simulink model "example_main_NDI_f16"  (R2020a)
settings: Solver=ode4  StartTime=0.0  StopTime=75  FixedStep=0.01  RelTol=1e-3
PreLoadFcn:
  | PreLoadFcn
values from neighbouring files (symbols this model uses):
  g = 32.17    [PreLoadFcn.m]
  N = [ 1      0     0.25 ... (first row only)    [PreLoadFcn.m]
  state0 = [IC.npos IC.epos IC.alt IC.q0 IC.q1 IC.q2 IC.q3  IC.p IC.q IC.r IC.alpha IC.beta IC.mu IC.Vt IC.chi IC.gamma]    [PreLoadFcn.m]
undefined symbols (not defined in the file or in its folder): Aactuator, ac, AeroCoeff, EngineTable, ft, IC, kg, m, Newton, PIController, Raphson, s, sigbuilder_block, slug
libraries: aerolibconvert2 x19, simulink x13, sharedutil x1
(part 2 of 6)

== system example_main_NDI_f16/Environment/ISP  ==
  note: 1 T
      | 2 a (Speed of sound)
      | 3 P
      | 4 rho
      | 5 g
      | 6 mu (Coefficient of viscosity)
  In Bus Element : Inport  PortName=PlantData  Element=Vt
  In Bus Element1 : Inport  PortName=PlantData  Element=altitude
  Demux : Demux  Outputs=[1,1,1,1,1,1]
      settings: DisplayOption=none
  Density Conversion : aerolibconvert2/Density Conversion  IU=kg/m^3  OU=slug/ft^3
      settings: SourceProductBaseCode=AE
  Divide1 : Product  Inputs=*/
  Length Conversion : aerolibconvert2/Length Conversion  IU=ft  OU=m
  MATLAB Function : MATLAB Function  TreatAsAtomicUnit=on
  Product : Product
  Square : Math  Operator=square  SignedPower=on  SaturateOnIntegerOverflow=on
  Velocity Conversion : aerolibconvert2/Velocity Conversion  IU=m/s  OU=ft/s
  r2d1 : Gain  Gain=0.5  SaturateOnIntegerOverflow=on  OutDataTypeStr=Inherit: Same as input  ParamDataTypeStr=Inherit: Same as input
  r2d2 : Gain  Gain=-1  SaturateOnIntegerOverflow=on  OutDataTypeStr=Inherit: Same as input  ParamDataTypeStr=Inherit: Same as input
  P(HPa) : Outport  VectorParamsAs1DForOutWhenUnconnected=off
  rho(kg/m^3) : Outport  Port=2  VectorParamsAs1DForOutWhenUnconnected=off
  qbar (lbf/ft^2) : Outport  Port=3  VectorParamsAs1DForOutWhenUnconnected=off
  "Mach " : Outport  Port=4  VectorParamsAs1DForOutWhenUnconnected=off
  T(K) : Outport  Port=5  VectorParamsAs1DForOutWhenUnconnected=off
  g (m/s^2) : Outport  Port=6  VectorParamsAs1DForOutWhenUnconnected=off
  mu : Outport  Port=7  VectorParamsAs1DForOutWhenUnconnected=off
  wires:
  MATLAB Function/1(ISP_output) -> Demux/1
  Length Conversion/1 -> MATLAB Function/1(h)
  Velocity Conversion/1 -> Divide1/2
  Density Conversion/1 -> Product/2  "rho(slugs/ft^3)"
  Demux/4 -> Density Conversion/1, rho(kg/m^3)/1  "rho(kg/m^3)"
  Demux/2 -> Velocity Conversion/1  "a(m/s)"
  Demux/1 -> T(K)/1  "T(K)"
  Divide1/1 -> "Mach "/1
  Demux/5 -> g (m/s^2)/1  "g (m/s^2)"
  Demux/6 -> mu/1  "mu"
  Product/1 -> r2d1/1
  Square/1 -> Product/1
  In Bus Element/1 -> Divide1/1, Square/1  "Vt (ft/s)"
  Demux/3 -> P(HPa)/1  "P(Pa)"
  r2d2/1 -> Length Conversion/1  "H(ft)"
  r2d1/1 -> qbar (lbf/ft^2)/1  "qbar (lbf/ft^2)"
  In Bus Element1/1 -> r2d2/1

== system example_main_NDI_f16/F-16 Vehicle Systems Model/6.4.3加裝向量噴嘴以及減速版打開30度模擬著陸速度為200， 上下偏轉向量噴嘴權重值為4，75S (附錄B須調整權重值: 2、4、8、16) ==
  Demux : Demux  Tag=STV Demux  Outputs=5
      settings: DisplayOption=none
  FromWs : FromWorkspace  Tag=STV FromWs  VariableName=tuvar
      SigBuilderData=|
      | common.afterFinalStr = 'Extrapolate'
      | common.sampleTime = 0
      | dataSet.timeRange = [0 90]
      | dataSet.name = 'Group 1'
      | sbobj.Groups.Name = 'Group 1'
      | sbobj.Groups.Signals(1).Name = 'Vt (ft/s)'
      | sbobj.Groups.Signals(1).XData = [0 5 6.2 7.35 8.3 9.05 10.05 11.2 13.1 14.75 15 16.85 18.75 19.63 20 22.2 23.5 25 26.65 30 31.65 40 50 60 75 80 90]
      | sbobj.Groups.Signals(1).YData = [287 287 286.6 286 285 284.6 283.9 283.4 281.8 279.8 279.4 277 274.8 273.8 273.3 270.3 268.6 266.55 263.7 260 258 250 240 227 200 226 210]
      | sbobj.Groups.Signals(2).Name = 'y (ft)'
      | sbobj.Groups.Signals(2).XData = [0 90]
      | sbobj.Groups.Signals(2).YData = [0 0]
      | sbobj.Groups.Signals(3).Name = 'h (ft)'
      | sbobj.Groups.Signals(3).XData = [0 55 75 90]
      | sbobj.Groups.Signals(3).YData = [993 93 0 0]
      | sbobj.Groups.Signals(4).Name = 'speed brake (deg)'
      | sbobj.Groups.Signals(4).XData = [0 90]
      | sbobj.Groups.Signals(4).YData = [30 30]
      | sbobj.Groups.Signals(5).Name = 'LandingGear_position'
      | sbobj.Groups.Signals(5).XData = [0 90]
      | sbobj.Groups.Signals(5).YData = [1 1]
      | sbobj.Groups.TimeRange = [0 90]
  Vt (ft/s) : Outport  Tag=STV Outport  VectorParamsAs1DForOutWhenUnconnected=off
  y (ft) : Outport  Tag=STV Outport  Port=2  VectorParamsAs1DForOutWhenUnconnected=off
  h (ft) : Outport  Tag=STV Outport  Port=3  VectorParamsAs1DForOutWhenUnconnected=off
  speed brake (deg) : Outport  Tag=STV Outport  Port=4
  LandingGear_position : Outport  Tag=STV Outport  Port=5
  wires:
  FromWs/1 -> Demux/1
  Demux/1 -> Vt (ft/s)/1
  Demux/2 -> y (ft)/1
  Demux/3 -> h (ft)/1
  Demux/4 -> speed brake (deg)/1
  Demux/5 -> LandingGear_position/1

== system example_main_NDI_f16/F-16 Vehicle Systems Model/6.4.3加裝向量噴嘴以及減速版打開40度模擬著陸速度為200， 上下偏轉向量噴嘴權重值為5.5，75S ==
  Demux : Demux  Tag=STV Demux  Outputs=5
      settings: DisplayOption=none
  FromWs : FromWorkspace  Tag=STV FromWs  VariableName=tuvar
      SigBuilderData=|
      | common.afterFinalStr = 'Extrapolate'
      | common.sampleTime = 0
      | dataSet.timeRange = [0 80]
      | dataSet.name = 'Group 1'
      | sbobj.Groups.Name = 'Group 1'
      | sbobj.Groups.Signals(1).Name = 'Vt (ft/s)'
      | sbobj.Groups.Signals(1).XData = [0 5 6.2 7.35 8.3 9.05 10.05 11.2 13.1 14.75 15 16.85 18.75 19.63 20 22.2 23.5 25 26.65 33 36.65 45 55 65 75 80]
      | sbobj.Groups.Signals(1).YData = [287 287 286.6 286 285 284.6 283.9 283.4 281.8 279.8 279.4 277 274.8 273.8 273.3 270.3 268.6 266.55 264 258 255.5 246 234 220 200 214]
      | sbobj.Groups.Signals(2).Name = 'y (ft)'
      | sbobj.Groups.Signals(2).XData = [0 80]
      | sbobj.Groups.Signals(2).YData = [0 0]
      | sbobj.Groups.Signals(3).Name = 'h (ft)'
      | sbobj.Groups.Signals(3).XData = [0 55 75 80]
      | sbobj.Groups.Signals(3).YData = [993 93 0 0]
      | sbobj.Groups.Signals(4).Name = 'speed brake (deg)'
      | sbobj.Groups.Signals(4).XData = [0 80]
      | sbobj.Groups.Signals(4).YData = [40 40]
      | sbobj.Groups.Signals(5).Name = 'LandingGear_position'
      | sbobj.Groups.Signals(5).XData = [0 80]
      | sbobj.Groups.Signals(5).YData = [1 1]
      | sbobj.Groups.TimeRange = [0 80]
  Vt (ft/s) : Outport  Tag=STV Outport  VectorParamsAs1DForOutWhenUnconnected=off
  y (ft) : Outport  Tag=STV Outport  Port=2  VectorParamsAs1DForOutWhenUnconnected=off
  h (ft) : Outport  Tag=STV Outport  Port=3  VectorParamsAs1DForOutWhenUnconnected=off
  speed brake (deg) : Outport  Tag=STV Outport  Port=4  VectorParamsAs1DForOutWhenUnconnected=off
  LandingGear_position : Outport  Tag=STV Outport  Port=5  VectorParamsAs1DForOutWhenUnconnected=off
  wires:
  FromWs/1 -> Demux/1
  Demux/1 -> Vt (ft/s)/1
  Demux/2 -> y (ft)/1
  Demux/3 -> h (ft)/1
  Demux/4 -> speed brake (deg)/1
  Demux/5 -> LandingGear_position/1

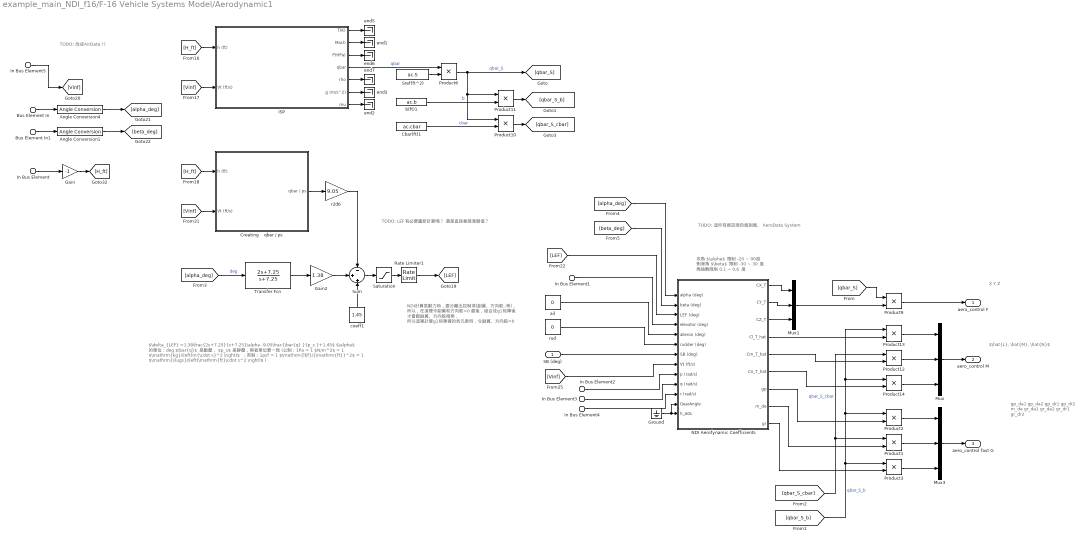
== system example_main_NDI_f16/F-16 Vehicle Systems Model/Aerodynamic1 ==
  note: NDI計算氣動力時，要分離出控制項(副翼、方向舵..等)，
      | 所以，在這裡令副翼和方向舵=0
      | 最後，組合成g1矩陣後 才會跟副翼、方向舵相乘，
      | 所以這裡計算g1矩陣裡的各元素時，令副翼、方向舵=0
  note: TODO: LEF有必要重新計算嗎？
      | 還是直接拿感測器值？
  note: X
      | Y
      | Z
  note: gp_da1
      | gp_da2
      | gp_dr1
      | gp_dr2
      | m_de
      | gr_da1
      | gr_da2
      | gr_dr1
      | gr_dr2
  note: $\delta_{LEF} =1.38\frac{2s+7.25}{s+7.25}\alpha -9.05\frac{\bar{q} }{p_s }+1.45$
      | $\alpha$ 的單位：deg
      | $\bar{q}$ 是動壓， $p_s$ 是靜壓，兩者單位要一致 (公制：1Pa = 1 $N/m^2$ = 1 $\mathrm{kg}/\left(m{\cdot s}^2 \right)$ ；英制：1psf = 1 $\mathrm{lbf}/{\mathrm{ft}}^2$ = 1 $\mathrm{slugs}/\left(\mathrm{ft}\cdot s^2 \right)$ )
  note: $\hat{L}, \hat{M}, \hat{N}$
  note: TODO: 這所有資訊源自感測器、
      | AeroData System
  note: TODO: 改成AirData !?
  note: 攻角 $\alpha$ 限制 -20 ~ 90度
      | 側滑角 $\beta$ 限制 -30 ~ 30 度
      | 馬赫數限制 0.1 ~ 0.6 度
  SB (deg) : Inport  Unit=deg
  In Bus Element : Inport  Port=2  PortName=PlantData  Element=altitude
  In Bus Element1 : Inport  Port=2  PortName=PlantData  Element=AeroActBus.Elevator_deg
  In Bus Element2 : Inport  Port=2  PortName=PlantData  Element=p
  In Bus Element3 : Inport  Port=2  PortName=PlantData  Element=q
  In Bus Element4 : Inport  Port=2  PortName=PlantData  Element=r
  In Bus Element5 : Inport  Port=2  PortName=PlantData  Element=Vt
  Bus Element In : Inport  Port=3  PortName=AirData  Element=alpha
  Bus Element In1 : Inport  Port=3  PortName=AirData  Element=beta
  Angle Conversion1 : aerolibconvert2/Angle Conversion  IU=rad  OU=deg
  Angle Conversion4 : aerolibconvert2/Angle Conversion  IU=rad  OU=deg
  Cbar(ft)1 : Constant  Value=ac.cbar
  Creating    qbar / ps : Subsystem
  Gain : Gain  Gain=-1
  Gain2 : Gain  Gain=1.38  SaturateOnIntegerOverflow=on  OutDataTypeStr=Inherit: Same as input  ParamDataTypeStr=Inherit: Same as input
  Ground : Ground
  "ISP " : Subsystem
  Mux : Mux  Inputs=3
  Mux1 : Mux  Inputs=3
  Mux3 : Mux  Inputs=3
  NDI Aerofynamic Coefficients : Subsystem
  Product{1..3,6,9..14} (10 alike) : Product
  Rate Limiter1 : RateLimiter  RisingSlewLimit=Aactuator.LEF.RateLimitUpper  FallingSlewLimit=Aactuator.LEF.RateLimitLower  SampleTimeMode=inherited  InitialCondition=Aactuator.LEF.IntegratorInitial
  Saturation : Saturate  UpperLimit=Aactuator.LEF.AngleLimitUpper  LowerLimit=Aactuator.LEF.AngleLimitLower
  Sref(ft^2) : Constant  Value=ac.S
  Sum : Sum  Inputs=-|+|+  InputSameDT=on  SaturateOnIntegerOverflow=on  OutDataTypeStr=Inherit: Same as first input
  Transfer Fcn : TransferFcn  Numerator=[2 7.25]  Denominator=[1 7.25]
  ail : Constant  Value=0
  b(ft)1 : Constant  Value=ac.b
  coeff1 : Constant  Value=1.45
  end{1..3,5..7} (6 alike) : Terminator
  r2d6 : Gain  Gain=9.05  SaturateOnIntegerOverflow=on  OutDataTypeStr=Inherit: Same as input  ParamDataTypeStr=Inherit: Same as input
  rud : Constant  Value=0
  aero_control F : Outport  VectorParamsAs1DForOutWhenUnconnected=off
  aero_control M : Outport  Port=2  VectorParamsAs1DForOutWhenUnconnected=off
  aero_control fast G : Outport  Port=3  VectorParamsAs1DForOutWhenUnconnected=off
  wires:
  [Vinf] -> "ISP "/2(Vt (ft/s))
  "ISP "/2("Mach ") -> end1/1
  "ISP "/7(mu) -> end2/1
  "ISP "/6(g (m/s^2)) -> end3/1
  "ISP "/5(rho) -> end7/1
  "ISP "/4("qbar ") -> Product6/1  "qbar"
  "ISP "/3(P(HPa)) -> end6/1
  "ISP "/1(T(K)) -> end5/1
  r2d6/1 -> Sum/1
  Creating    qbar / ps/1(qbar / ps) -> r2d6/1
  [alpha_deg] -> Transfer Fcn/1  "deg"
  [Vinf] -> Creating    qbar / ps/2(Vt (ft/s))
  coeff1/1 -> Sum/3
  [H_ft] -> Creating    qbar / ps/1(h (ft))
  [H_ft] -> "ISP "/1(h (ft))
  Sum/1 -> Saturation/1
  Saturation/1 -> Rate Limiter1/1
  Rate Limiter1/1 -> [LEF]
  Transfer Fcn/1 -> Gain2/1
  In Bus Element/1 -> Gain/1
  Gain/1 -> [H_ft]
  Cbar(ft)1/1 -> Product10/2  "cbar"
  b(ft)1/1 -> Product11/2  "b"
  Sref(ft^2)/1 -> Product6/2
  Product10/1 -> [qbar_S_cbar]
  Product6/1 -> Product11/1, Product10/1, [qbar_S]  "qbar_S"
  Product11/1 -> [qbar_S_b]
  [qbar_S] -> Product9/1
  Product9/1 -> aero_control F/1
  Product12/1 -> Mux/2
  Product13/1 -> Mux/1
  Product14/1 -> Mux/3
  Mux/1 -> aero_control M/1
  NDI Aerofynamic Coefficients/4(Cl_T_hat) -> Product13/2
  NDI Aerofynamic Coefficients/5(Cm_T_hat) -> Product12/2
  NDI Aerofynamic Coefficients/6(Cn_T_hat) -> Product14/2
  NDI Aerofynamic Coefficients/1(CX_T) -> Mux1/1
  NDI Aerofynamic Coefficients/2(CY_T) -> Mux1/2
  NDI Aerofynamic Coefficients/3(CZ_T) -> Mux1/3
  Mux1/1 -> Product9/2
  [qbar_S_b] -> Product13/1, Product14/1, Product2/1, Product3/1  "qbar_S_b"
  Product3/1 -> Mux3/3
  Product1/1 -> Mux3/2
  Product2/1 -> Mux3/1
  NDI Aerofynamic Coefficients/7(gp) -> Product2/2
  [qbar_S_cbar] -> Product12/1, Product1/1  "qbar_S_cbar"
  NDI Aerofynamic Coefficients/9(gr) -> Product3/2
  NDI Aerofynamic Coefficients/8(m_de) -> Product1/2
  Mux3/1 -> aero_control fast G/1
  [Vinf] -> NDI Aerofynamic Coefficients/8(Vt (ft/s))
  SB (deg)/1 -> NDI Aerofynamic Coefficients/7(SB (deg))
  [LEF] -> NDI Aerofynamic Coefficients/3(LEF (deg))
  rud/1 -> NDI Aerofynamic Coefficients/6(rudder (deg))
  ail/1 -> NDI Aerofynamic Coefficients/5(alieron (deg))
  In Bus Element1/1 -> NDI Aerofynamic Coefficients/4(elevator (deg))
  [beta_deg] -> NDI Aerofynamic Coefficients/2(beta (deg))
  [alpha_deg] -> NDI Aerofynamic Coefficients/1(alpha (deg))
  In Bus Element2/1 -> NDI Aerofynamic Coefficients/9(p (rad/s))
  In Bus Element3/1 -> NDI Aerofynamic Coefficients/10(q (rad/s))
  In Bus Element4/1 -> NDI Aerofynamic Coefficients/11(r (rad/s))
  Ground/1 -> NDI Aerofynamic Coefficients/12(GearAngle), NDI Aerofynamic Coefficients/13(h_AGL)
  Gain2/1 -> Sum/2
  Bus Element In/1 -> Angle Conversion4/1
  Angle Conversion4/1 -> [alpha_deg]
  Angle Conversion1/1 -> [beta_deg]
  Bus Element In1/1 -> Angle Conversion1/1
  In Bus Element5/1 -> [Vinf]

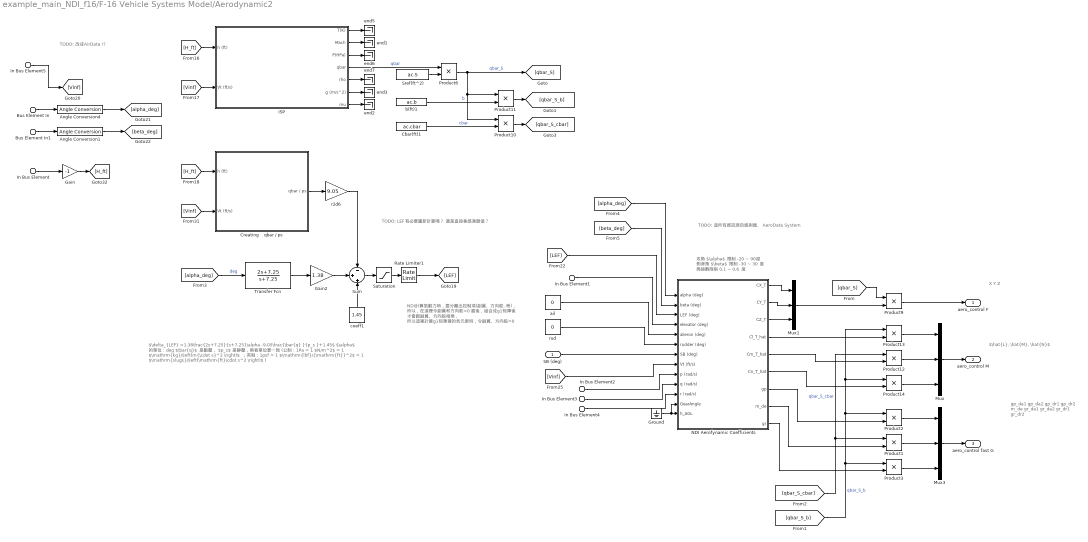
== system example_main_NDI_f16/F-16 Vehicle Systems Model/Aerodynamic2 ==
  note: NDI計算氣動力時，要分離出控制項(副翼、方向舵..等)，
      | 所以，在這裡令副翼和方向舵=0
      | 最後，組合成g1矩陣後 才會跟副翼、方向舵相乘，
      | 所以這裡計算g1矩陣裡的各元素時，令副翼、方向舵=0
  note: TODO: LEF有必要重新計算嗎？
      | 還是直接拿感測器值？
  note: X
      | Y
      | Z
  note: gp_da1
      | gp_da2
      | gp_dr1
      | gp_dr2
      | m_de
      | gr_da1
      | gr_da2
      | gr_dr1
      | gr_dr2
  note: $\delta_{LEF} =1.38\frac{2s+7.25}{s+7.25}\alpha -9.05\frac{\bar{q} }{p_s }+1.45$
      | $\alpha$ 的單位：deg
      | $\bar{q}$ 是動壓， $p_s$ 是靜壓，兩者單位要一致 (公制：1Pa = 1 $N/m^2$ = 1 $\mathrm{kg}/\left(m{\cdot s}^2 \right)$ ；英制：1psf = 1 $\mathrm{lbf}/{\mathrm{ft}}^2$ = 1 $\mathrm{slugs}/\left(\mathrm{ft}\cdot s^2 \right)$ )
  note: $\hat{L}, \hat{M}, \hat{N}$
  note: TODO: 這所有資訊源自感測器、
      | AeroData System
  note: TODO: 改成AirData !?
  note: 攻角 $\alpha$ 限制 -20 ~ 90度
      | 側滑角 $\beta$ 限制 -30 ~ 30 度
      | 馬赫數限制 0.1 ~ 0.6 度
  SB (deg) : Inport  Unit=deg
  In Bus Element : Inport  Port=2  PortName=PlantData  Element=altitude
  In Bus Element1 : Inport  Port=2  PortName=PlantData  Element=AeroActBus.Elevator_deg
  In Bus Element2 : Inport  Port=2  PortName=PlantData  Element=p
  In Bus Element3 : Inport  Port=2  PortName=PlantData  Element=q
  In Bus Element4 : Inport  Port=2  PortName=PlantData  Element=r
  In Bus Element5 : Inport  Port=2  PortName=PlantData  Element=Vt
  Bus Element In : Inport  Port=3  PortName=AirData  Element=alpha_c
  Bus Element In1 : Inport  Port=3  PortName=AirData  Element=beta_c
  Angle Conversion1 : aerolibconvert2/Angle Conversion  IU=rad  OU=deg
  Angle Conversion4 : aerolibconvert2/Angle Conversion  IU=rad  OU=deg
  Cbar(ft)1 : Constant  Value=ac.cbar
  Creating    qbar / ps : Subsystem
  Gain : Gain  Gain=-1
  Gain2 : Gain  Gain=1.38  SaturateOnIntegerOverflow=on  OutDataTypeStr=Inherit: Same as input  ParamDataTypeStr=Inherit: Same as input
  Ground : Ground
  "ISP " : Subsystem
  Mux : Mux  Inputs=3
  Mux1 : Mux  Inputs=3
  Mux3 : Mux  Inputs=3
  NDI Aerofynamic Coefficients : Subsystem
  Product{1..3,6,9..14} (10 alike) : Product
  Rate Limiter1 : RateLimiter  RisingSlewLimit=Aactuator.LEF.RateLimitUpper  FallingSlewLimit=Aactuator.LEF.RateLimitLower  SampleTimeMode=inherited  InitialCondition=Aactuator.LEF.IntegratorInitial
  Saturation : Saturate  UpperLimit=Aactuator.LEF.AngleLimitUpper  LowerLimit=Aactuator.LEF.AngleLimitLower
  Sref(ft^2) : Constant  Value=ac.S
  Sum : Sum  Inputs=-|+|+  InputSameDT=on  SaturateOnIntegerOverflow=on  OutDataTypeStr=Inherit: Same as first input
  Transfer Fcn : TransferFcn  Numerator=[2 7.25]  Denominator=[1 7.25]
  ail : Constant  Value=0
  b(ft)1 : Constant  Value=ac.b
  coeff1 : Constant  Value=1.45
  end{1..3,5..7} (6 alike) : Terminator
  r2d6 : Gain  Gain=9.05  SaturateOnIntegerOverflow=on  OutDataTypeStr=Inherit: Same as input  ParamDataTypeStr=Inherit: Same as input
  rud : Constant  Value=0
  aero_control F : Outport  VectorParamsAs1DForOutWhenUnconnected=off
  aero_control M : Outport  Port=2  VectorParamsAs1DForOutWhenUnconnected=off
  aero_control fast G : Outport  Port=3  VectorParamsAs1DForOutWhenUnconnected=off
  wires:
  [Vinf] -> "ISP "/2(Vt (ft/s))
  "ISP "/2("Mach ") -> end1/1
  "ISP "/7(mu) -> end2/1
  "ISP "/6(g (m/s^2)) -> end3/1
  "ISP "/5(rho) -> end7/1
  "ISP "/4("qbar ") -> Product6/1  "qbar"
  "ISP "/3(P(HPa)) -> end6/1
  "ISP "/1(T(K)) -> end5/1
  r2d6/1 -> Sum/1
  Creating    qbar / ps/1(qbar / ps) -> r2d6/1
  [alpha_deg] -> Transfer Fcn/1  "deg"
  [Vinf] -> Creating    qbar / ps/2(Vt (ft/s))
  coeff1/1 -> Sum/3
  [H_ft] -> Creating    qbar / ps/1(h (ft))
  [H_ft] -> "ISP "/1(h (ft))
  Sum/1 -> Saturation/1
  Saturation/1 -> Rate Limiter1/1
  Rate Limiter1/1 -> [LEF]
  Transfer Fcn/1 -> Gain2/1
  In Bus Element/1 -> Gain/1
  Gain/1 -> [H_ft]
  Cbar(ft)1/1 -> Product10/2  "cbar"
  b(ft)1/1 -> Product11/2  "b"
  Sref(ft^2)/1 -> Product6/2
  Product10/1 -> [qbar_S_cbar]
  Product6/1 -> Product11/1, Product10/1, [qbar_S]  "qbar_S"
  Product11/1 -> [qbar_S_b]
  [qbar_S] -> Product9/1
  Product9/1 -> aero_control F/1
  Product12/1 -> Mux/2
  Product13/1 -> Mux/1
  Product14/1 -> Mux/3
  Mux/1 -> aero_control M/1
  NDI Aerofynamic Coefficients/4(Cl_T_hat) -> Product13/2
  NDI Aerofynamic Coefficients/5(Cm_T_hat) -> Product12/2
  NDI Aerofynamic Coefficients/6(Cn_T_hat) -> Product14/2
  NDI Aerofynamic Coefficients/1(CX_T) -> Mux1/1
  NDI Aerofynamic Coefficients/2(CY_T) -> Mux1/2
  NDI Aerofynamic Coefficients/3(CZ_T) -> Mux1/3
  Mux1/1 -> Product9/2
  [qbar_S_b] -> Product13/1, Product14/1, Product2/1, Product3/1  "qbar_S_b"
  Product3/1 -> Mux3/3
  Product1/1 -> Mux3/2
  Product2/1 -> Mux3/1
  NDI Aerofynamic Coefficients/7(gp) -> Product2/2
  [qbar_S_cbar] -> Product12/1, Product1/1  "qbar_S_cbar"
  NDI Aerofynamic Coefficients/9(gr) -> Product3/2
  NDI Aerofynamic Coefficients/8(m_de) -> Product1/2
  Mux3/1 -> aero_control fast G/1
  [Vinf] -> NDI Aerofynamic Coefficients/8(Vt (ft/s))
  SB (deg)/1 -> NDI Aerofynamic Coefficients/7(SB (deg))
  [LEF] -> NDI Aerofynamic Coefficients/3(LEF (deg))
  rud/1 -> NDI Aerofynamic Coefficients/6(rudder (deg))
  ail/1 -> NDI Aerofynamic Coefficients/5(alieron (deg))
  In Bus Element1/1 -> NDI Aerofynamic Coefficients/4(elevator (deg))
  [beta_deg] -> NDI Aerofynamic Coefficients/2(beta (deg))
  [alpha_deg] -> NDI Aerofynamic Coefficients/1(alpha (deg))
  In Bus Element2/1 -> NDI Aerofynamic Coefficients/9(p (rad/s))
  In Bus Element3/1 -> NDI Aerofynamic Coefficients/10(q (rad/s))
  In Bus Element4/1 -> NDI Aerofynamic Coefficients/11(r (rad/s))
  Ground/1 -> NDI Aerofynamic Coefficients/12(GearAngle), NDI Aerofynamic Coefficients/13(h_AGL)
  Gain2/1 -> Sum/2
  Bus Element In/1 -> Angle Conversion4/1
  Angle Conversion4/1 -> [alpha_deg]
  Angle Conversion1/1 -> [beta_deg]
  Bus Element In1/1 -> Angle Conversion1/1
  In Bus Element5/1 -> [Vinf]

== system example_main_NDI_f16/F-16 Vehicle Systems Model/Iteration Algorithm V chi gamma ==
  note: $\mu_c ={\mathrm{tan}}^{-1} {\left(\frac{V_T {\chi^˙ }_{des} \mathrm{cos}\gamma }{V_T {\gamma^˙ }_{des} +g\mathrm{cos}\gamma }\right)}$
  note: $\alpha_c ={\mathrm{tan}}^{-1} {\left(\frac{-L+mV_T {\chi^˙ }_{des} \mathrm{cos}\gamma \mathrm{sin}\mu_c +mV_T {\gamma^˙ }_{des} \mathrm{cos}\mu_c +mg\mathrm{cos}\gamma \mathrm{cos}\mu_c }{m{\dot{V} }_{T_{des} } +D+mg\mathrm{sin}\gamma }\right)}$
  note: $T_c =\frac{1}{\mathrm{cos}\alpha_c }{\left(m{\dot{V} }_{T_{des} } +D+mg\mathrm{sin}\gamma \right)}$
  alpha_c : Inport
  aero F : Inport  Port=2
  Vt,chi,gamma dot desire : Inport  Port=3
  beta_cmd : Inport  Port=4
  gravity : Inport  Port=5
  In Bus Element4 : Inport  Port=6  PortName=AirData  Element=Vt
  In Bus Element5 : Inport  Port=6  PortName=AirData  Element=gamma
  Drag_c : Fcn  Expr=-u(4)*cos(u(2))*cos(u(3))-u(5)*sin(u(3))-u(6)*sin(u(2))*cos(u(3))
  Lift_c : Fcn  Expr=u(4)*sin(u(2))-u(6)*cos(u(2))
  Mux : Mux
  Mux1 : Mux
  Mux2 : Mux  Inputs=5
  Mux{3..6} (4 alike) : Mux  Inputs=2
  Mux7 : Mux  Inputs=5
  Saturation : Saturate  UpperLimit=deg2rad(80)  LowerLimit=deg2rad(-15)
  Thrust_c function1 : Fcn  Expr=(u(8)*u(1)+u(6)+u(8)*u(9)*sin(u(5)))/(cos(u(10)))
  To Workspace : ToWorkspace  VariableName=Drag_c_Lift_c  SaveFormat=Timeseries  SampleTime=-1
  alpha_c function2 : Fcn  Expr=atan2((-u(9)+u(10)*u(6)*cos(u(7))*sin(u(4))*u(2)+u(10)*u(6)*cos(u(4))*u(3)+u(10)*u(11)*cos(u(7))*cos(u(4))),(u(10)*u(1)+u(8)+u(10)*u(11)*sin(u(7))))
  mass (slugs) : Constant  Value=ac.m
  mu_c : Fcn  Expr=atan2((u(4)*u(2)*cos(u(5))),(u(4)*u(3)+u(6)*cos(u(5))))
  thrust_command : Outport  VectorParamsAs1DForOutWhenUnconnected=off
  mu_command : Outport  Port=2  VectorParamsAs1DForOutWhenUnconnected=off
  alpha_command : Outport  Port=3  VectorParamsAs1DForOutWhenUnconnected=off
  beta_command : Outport  Port=4  VectorParamsAs1DForOutWhenUnconnected=off
  wires:
  Vt,chi,gamma dot desire/1 -> Mux/1, Mux2/1, Mux7/1  "Vt,chi,gamma dot desire"
  In Bus Element4/1 -> Mux6/1, Mux1/1, Mux/2  "Vt"
  In Bus Element5/1 -> Mux6/2, Mux/3  "gamma"
  Mux/1 -> mu_c/1
  gravity/1 -> Mux/4, Mux5/2  "g"
  mu_c/1 -> Mux4/1, mu_command/1  "mu_c"
  aero F/1 -> Mux1/4  "X,Y,Z"
  beta_cmd/1 -> Mux4/2, Mux1/3, beta_command/1  "beta_c"
  alpha_c/1 -> Mux1/2  "alpha_c"
  Mux1/1 -> Drag_c/1, Lift_c/1
  Drag_c/1 -> Mux3/1  "Drag_c"
  Lift_c/1 -> Mux3/2  "Lift_c"
  Mux3/1 -> To Workspace/1, Mux7/3, Mux2/4  "Drag_c,Lift_c"
  Mux4/1 -> Mux2/2  "mu_c,beta_c"
  mass (slugs)/1 -> Mux5/1  "mass"
  Mux5/1 -> Mux2/5, Mux7/4  "mass,gravity"
  Mux6/1 -> Mux7/2, Mux2/3  "Vt,gamma"
  Mux2/1 -> alpha_c function2/1
  Mux7/1 -> Thrust_c function1/1
  Thrust_c function1/1 -> thrust_command/1  "thrust_c"
  alpha_c function2/1 -> Saturation/1  "alpha_c"
  Saturation/1 -> alpha_command/1, Mux7/5

== system example_main_NDI_f16/F-16 Vehicle Systems Model/Iteration Algorithm Y Z ==
  note: $\chi_c ={\mathrm{sin}}^{-1} {\left(\frac{{\dot{Y} }_{des} }{\sqrt{V_{T_c }^2 -{\dot{Z} }_{des}^2 }}\right)}$
  note: $\gamma_c =-{\mathrm{sin}}^{-1} {\left(\frac{{\dot{Z} }_{des} }{V_{T_c } }\right)}$
  Vc : Inport
  Ydot,Zdot des : Inport  Port=2
  Asin : Trigonometry  Operator=asin
  Asin1 : Trigonometry  Operator=asin
  Demux : Demux  Outputs=2
  Divide : Product  Inputs=*/
  Divide1 : Product  Inputs=*/
  Minus : Sum  Inputs=+-
  Multiply : Gain  Gain=-1
  Square : Math  Operator=square  SaturateOnIntegerOverflow=on
  Square Root : Sqrt  SaturateOnIntegerOverflow=on
  Square1 : Math  Operator=square  SaturateOnIntegerOverflow=on
  chi_c : Outport  VectorParamsAs1DForOutWhenUnconnected=off
  gamma_c : Outport  Port=2  VectorParamsAs1DForOutWhenUnconnected=off
  wires:
  Vc/1 -> Square/1, Divide/2  "Vc"
  Ydot,Zdot des/1 -> Demux/1
  Asin/1 -> Multiply/1
  Divide/1 -> Asin/1
  Demux/2 -> Square1/1, Divide/1  "Z_dot_desire"
  Demux/1 -> Divide1/1  "Y_dot_desire"
  Multiply/1 -> gamma_c/1
  Asin1/1 -> chi_c/1
  Divide1/1 -> Asin1/1
  Square Root/1 -> Divide1/2
  Square/1 -> Minus/1
  Square1/1 -> Minus/2
  Minus/1 -> Square Root/1

== system example_main_NDI_f16/F-16 Vehicle Systems Model/Vehicle ==
  note: 攻角 $\alpha$ 限制 -20 ~ 90度
      | 側滑角 $\beta$ 限制 -30 ~ 30 度
      | 馬赫數限制 0.1 ~ 0.6 度
  note: F-16 Nonlinear Model
  note: Tx
      | Ty
      | Tz
      | ---
      | Mx_T
      | My_T
      | Mz_T
  note: 高度限制 0 ~ 50000 ft
      | 馬赫數限制 0 ~ 1 馬赫
  fadec_cmd : Inport
  fcs_cmd : Inport  Port=2
  " SB_deg" : Inport  Port=3
  Bus Element In : Inport  Port=4  PortName=EnvData
  Bus Element In1 : Inport  Port=4  PortName=EnvData
  In Bus Element : Inport  Port=4  PortName=EnvData  Element=g
  6DOF (Quaternion) : Subsystem
  Actuators (no roll off)1 : Subsystem  Commented=on
  Aerodynamics : Subsystem
  Demux4 : Demux  Outputs=[3, 3]
  Demux5 : Demux  Outputs=[3, 3]
  ModelBus : BusCreator  Inputs=23
  Propulsion : Subsystem
  Sum : Sum  Inputs=|++
  Terminator2 : Terminator
  PlantData : Outport
  wires:
  6DOF (Quaternion)/4(q0q1q2q3) -> ModelBus/4
  6DOF (Quaternion)/11(Vt) -> ModelBus/11
  6DOF (Quaternion)/3(altitude) -> ModelBus/3
  ModelBus/1 -> Aerodynamics/4(PlantData), Propulsion/3(PlantData), PlantData/1  "PlantData"
  6DOF (Quaternion)/1(npos) -> ModelBus/1
  6DOF (Quaternion)/2(epos) -> ModelBus/2
  " SB_deg"/1 -> Aerodynamics/3(" SB (deg)")
  Aerodynamics/1(FM) -> Sum/2, 6DOF (Quaternion)/3(AeroFM)
  Aerodynamics/2(ActSensor_Out) -> [AeroActBus]
  Propulsion/1(FM) -> Demux5/1, Sum/1
  fcs_cmd/1 -> [fcs_cmd], Aerodynamics/2(fcs_cmd)  "fcs_cmd"
  fadec_cmd/1 -> Propulsion/2(fadec_cmd), [fadec_cmd]  "fadec_cmd"
  Propulsion/2(ActSensor_Out) -> [PropActBus]
  Propulsion/3(PropData) -> [PropBus]
  Sum/1 -> Demux4/1
  Demux4/2 -> 6DOF (Quaternion)/2(Mxyz)
  Demux4/1 -> 6DOF (Quaternion)/1(Fxyz)
  Demux5/1 -> 6DOF (Quaternion)/4(Txyz)
  Demux5/2 -> Terminator2/1
  In Bus Element/1 -> 6DOF (Quaternion)/5(gravity)
  6DOF (Quaternion)/17(an) -> ModelBus/17
  6DOF (Quaternion)/18(ay) -> ModelBus/18
  6DOF (Quaternion)/5(p) -> ModelBus/5
  6DOF (Quaternion)/6(q) -> ModelBus/6
  6DOF (Quaternion)/7(r) -> ModelBus/7
  6DOF (Quaternion)/8(alpha) -> ModelBus/8
  6DOF (Quaternion)/9(beta) -> ModelBus/9
  6DOF (Quaternion)/10(mu) -> ModelBus/10
  6DOF (Quaternion)/12(chi) -> ModelBus/12
  6DOF (Quaternion)/13(gamma) -> ModelBus/13
  6DOF (Quaternion)/14(phi) -> ModelBus/14
  6DOF (Quaternion)/15(theta) -> ModelBus/15
  6DOF (Quaternion)/16(psi) -> ModelBus/16
  Bus Element In/1 -> Aerodynamics/1(EnvData)
  Bus Element In1/1 -> Propulsion/1(EnvData)
  [PropActBus] -> ModelBus/21  "PropActBus"
  [AeroActBus] -> ModelBus/19  "AeroActBus"
  [PropBus] -> ModelBus/20  "PropBus"
  [fadec_cmd] -> ModelBus/22
  [fcs_cmd] -> ModelBus/23

== system example_main_NDI_f16/F-16 Vehicle Systems Model/pqr NDI Controller ==
  note: 1) Add Subsystem or Model blocks as valid variant choices.
      | 2) You cannot connect blocks at this level. At simulation, connectivity is automatically
      | determined, based on the active variant and port name matching.
  coef M : Inport
  control g : Inport  Port=2
  pqr dot desire : Inport  Port=3
  PlantData : Inport  Port=4
  AirData : Inport  Port=5
  p q r : Inport  Port=6
  TVC OFF : Subsystem  VariantControl=TVC OFF
  TVC ON : Subsystem  VariantControl=TVC ON
  TVC_z : Outport
  "TVC_y " : Outport  Port=2
  elevator : Outport  Port=3
  aileron : Outport  Port=4
  rudder : Outport  Port=5

== system example_main_NDI_f16/F-16 Vehicle Systems Model/μαβ NDI Controller ==
  aero F : Inport
  μαβ dot desire : Inport  Port=2
  gravity : Inport  Port=3
  In Bus Element : Inport  Port=4  PortName=PlantData  Element=PropBus.T
  In Bus Element2 : Inport  Port=5  PortName=AirData  Element=alpha
  In Bus Element4 : Inport  Port=5  PortName=AirData  Element=alpha
  In Bus Element3 : Inport  Port=5  PortName=AirData  Element=beta
  In Bus Element5 : Inport  Port=5  PortName=AirData  Element=beta
  In Bus Element6 : Inport  Port=5  PortName=AirData  Element=mu
  In Bus Element7 : Inport  Port=5  PortName=AirData  Element=Vt
  In Bus Element8 : Inport  Port=5  PortName=AirData  Element=gamma
  Mux : Mux  Inputs=5
  Sum : Sum  Inputs=+-|
  attitude NDI : MATLAB Function  TreatAsAtomicUnit=on
  command matrix (5.5.4) : Subsystem
  f2 (5.5.3) : Subsystem
  pc : Outport  VectorParamsAs1DForOutWhenUnconnected=off
  qc : Outport  Port=2  VectorParamsAs1DForOutWhenUnconnected=off
  rc : Outport  Port=3  VectorParamsAs1DForOutWhenUnconnected=off
  D : Outport  Port=4  VectorParamsAs1DForOutWhenUnconnected=off
  Y : Outport  Port=5  VectorParamsAs1DForOutWhenUnconnected=off
  L : Outport  Port=6  VectorParamsAs1DForOutWhenUnconnected=off
  wires:
  f2 (5.5.3)/1(f2) -> Sum/2
  μαβ dot desire/1 -> Sum/1
  Sum/1 -> attitude NDI/1(y_bar)
  attitude NDI/1(p_c) -> pc/1
  attitude NDI/2(q_c) -> qc/1
  attitude NDI/3(r_c) -> rc/1
  command matrix (5.5.4)/1(g2) -> attitude NDI/2(g2)
  Mux/1 -> f2 (5.5.3)/1(aero V)  "V, α, β, μ, γ"
  In Bus Element/1 -> f2 (5.5.3)/4(Thrust)
  aero F/1 -> f2 (5.5.3)/2(X,Y,Z)
  f2 (5.5.3)/2(D) -> D/1
  f2 (5.5.3)/3(Y) -> Y/1
  f2 (5.5.3)/4(L) -> L/1
  gravity/1 -> f2 (5.5.3)/3(gravity)
  In Bus Element2/1 -> command matrix (5.5.4)/1(α)
  In Bus Element3/1 -> command matrix (5.5.4)/2(β)
  In Bus Element5/1 -> Mux/3
  In Bus Element4/1 -> Mux/2
  In Bus Element6/1 -> Mux/4
  In Bus Element7/1 -> Mux/1
  In Bus Element8/1 -> Mux/5

== system example_main_NDI_f16/F-16 Vehicle Systems Model/Aerodynamic1/Creating    qbar // ps ==
  h (ft) : Inport
  Vt (ft/s) : Inport  Port=2
  Constant2 : Constant
  Constant3 : Constant  Value=390
  Constant6 : Constant  Value=4.14
  Math Function : Math  Operator=pow  SignedPower=on  SaturateOnIntegerOverflow=on
  Math Function1 : Math  Operator=square  SignedPower=on  SaturateOnIntegerOverflow=on
  Product : Product  Inputs=/*  InputSameDT=on  SaturateOnIntegerOverflow=on  OutDataTypeStr=Inherit: Same as first input
  Product5 : Product  Inputs=**  InputSameDT=on  SaturateOnIntegerOverflow=on  OutDataTypeStr=Inherit: Same as first input
  Product6 : Product  Inputs=**  InputSameDT=on  SaturateOnIntegerOverflow=on  OutDataTypeStr=Inherit: Same as first input
  Sum3 : Sum  Inputs=+-|  InputSameDT=on  SaturateOnIntegerOverflow=on  OutDataTypeStr=Inherit: Same as first input
  Switch : Switch  Threshold=35000  SaturateOnIntegerOverflow=on  InputSameDT=on
  r2d2 : Gain  Gain=0.703e-5  SaturateOnIntegerOverflow=on  OutDataTypeStr=Inherit: Same as input  ParamDataTypeStr=Inherit: Same as input
  r2d3 : Gain  Gain=519  SaturateOnIntegerOverflow=on  OutDataTypeStr=Inherit: Same as input  ParamDataTypeStr=Inherit: Same as input
  r2d4 : Gain  Gain=0.5  SaturateOnIntegerOverflow=on  OutDataTypeStr=Inherit: Same as input  ParamDataTypeStr=Inherit: Same as input
  r2d5 : Gain  Gain=1715  SaturateOnIntegerOverflow=on  OutDataTypeStr=Inherit: Same as input  ParamDataTypeStr=Inherit: Same as input
  rho0 : Gain  Gain=2.377e-3  SaturateOnIntegerOverflow=on  OutDataTypeStr=Inherit: Same as input  ParamDataTypeStr=Inherit: Same as input
  qbar / ps : Outport  VectorParamsAs1DForOutWhenUnconnected=off
  wires:
  h (ft)/1 -> r2d2/1, Switch/2
  Sum3/1 -> Math Function/1, r2d3/1  "tfac"
  Constant3/1 -> Switch/1
  r2d3/1 -> Switch/3
  Constant6/1 -> Math Function/2
  rho0/1 -> Product5/1, Product6/2  "rho"
  r2d2/1 -> Sum3/2
  Constant2/1 -> Sum3/1
  Math Function/1 -> rho0/1
  Math Function1/1 -> Product5/2
  Switch/1 -> r2d5/1  "temp"
  r2d5/1 -> Product6/1
  Product6/1 -> Product/1  "ps"
  Product5/1 -> r2d4/1  "qbar"
  Product/1 -> qbar / ps/1
  Vt (ft/s)/1 -> Math Function1/1  "Vt (ft/s)"
  r2d4/1 -> Product/2

== system example_main_NDI_f16/F-16 Vehicle Systems Model/Aerodynamic1/ISP  ==
  note: 1 T
      | 2 a (Speed of sound)
      | 3 P
      | 4 rho
      | 5 g
      | 6 mu (Coefficient of viscosity)
  h (ft) : Inport
  Vt (ft/s) : Inport  Port=2
  Demux : Demux  Outputs=[1,1,1,1,1,1]
      settings: DisplayOption=none
  Divide1 : Product  Inputs=*/
  Length Conversion : aerolibconvert2/Length Conversion  IU=ft  OU=m
  MATLAB Function : MATLAB Function  TreatAsAtomicUnit=on
  Product : Product
  Square : Math  Operator=square  SignedPower=on  SaturateOnIntegerOverflow=on
  r2d1 : Gain  Gain=0.5  SaturateOnIntegerOverflow=on  OutDataTypeStr=Inherit: Same as input  ParamDataTypeStr=Inherit: Same as input
  r2d3 : Gain  Gain=3.2808399  SaturateOnIntegerOverflow=on  OutDataTypeStr=Inherit: Same as input  ParamDataTypeStr=Inherit: Same as input
  r2d4 : Gain  Gain=0.00194032033  SaturateOnIntegerOverflow=on  OutDataTypeStr=Inherit: Same as input  ParamDataTypeStr=Inherit: Same as input
  T(K) : Outport  VectorParamsAs1DForOutWhenUnconnected=off
  "Mach " : Outport  Port=2  VectorParamsAs1DForOutWhenUnconnected=off
  P(HPa) : Outport  Port=3  VectorParamsAs1DForOutWhenUnconnected=off
  "qbar " : Outport  Port=4  VectorParamsAs1DForOutWhenUnconnected=off
  rho : Outport  Port=5  VectorParamsAs1DForOutWhenUnconnected=off
  g (m/s^2) : Outport  Port=6  VectorParamsAs1DForOutWhenUnconnected=off
  mu : Outport  Port=7  VectorParamsAs1DForOutWhenUnconnected=off
  wires:
  r2d3/1 -> Divide1/2
  r2d1/1 -> Product/2
  Demux/4 -> rho/1, r2d4/1  "rho(kg/m^3)"
  Demux/2 -> r2d3/1  "a(m/s)"
  Demux/1 -> T(K)/1  "T(K)"
  r2d4/1 -> r2d1/1
  Divide1/1 -> "Mach "/1
  Demux/5 -> g (m/s^2)/1  "g (m/s^2)"
  Demux/6 -> mu/1  "mu"
  Product/1 -> "qbar "/1
  Square/1 -> Product/1
  Vt (ft/s)/1 -> Square/1, Divide1/1
  Demux/3 -> P(HPa)/1  "P(Pa)"
  h (ft)/1 -> Length Conversion/1
  Length Conversion/1 -> MATLAB Function/1(h)
  MATLAB Function/1(ISP_output) -> Demux/1

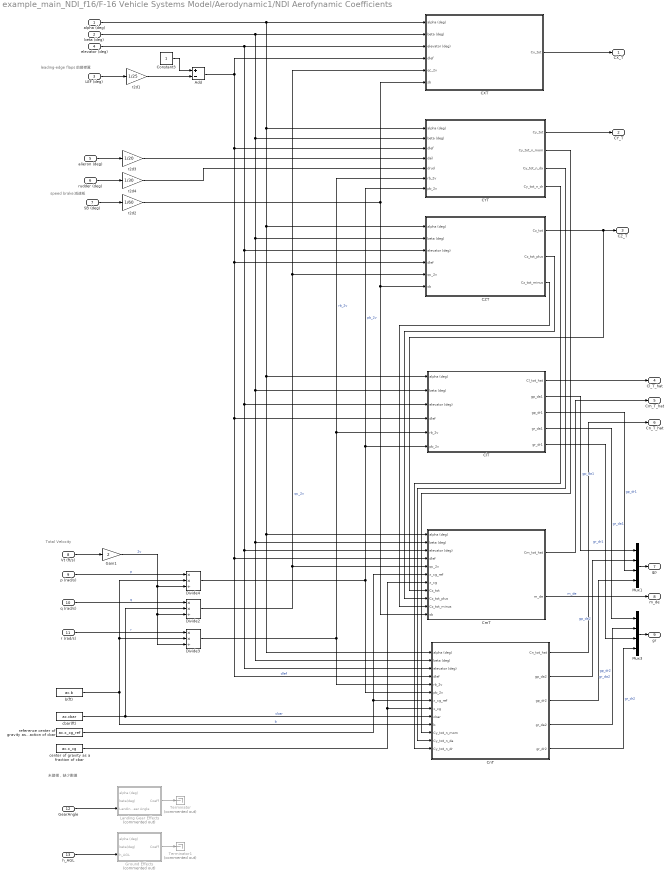
== system example_main_NDI_f16/F-16 Vehicle Systems Model/Aerodynamic1/NDI Aerofynamic Coefficients ==
  note: leading-edge flaps
      | 前緣襟翼
  note: speed brake
      | 減速板
  note: Total Velocity
  note: 未建模，缺少數據
  alpha (deg) : Inport
  beta (deg) : Inport  Port=2
  LEF (deg) : Inport  Port=3
  elevator (deg) : Inport  Port=4
  alieron (deg) : Inport  Port=5
  rudder (deg) : Inport  Port=6
  SB (deg) : Inport  Port=7  Unit=deg
  Vt (ft/s) : Inport  Port=8
  p (rad/s) : Inport  Port=9
  q (rad/s) : Inport  Port=10
  r (rad/s) : Inport  Port=11
  GearAngle : Inport  Port=12
  h_AGL : Inport  Port=13
  Add : Sum  Inputs=+-
  CXT : Subsystem
  CYT : Subsystem
  CZT : Subsystem
  ClT : Subsystem
  CmT : Subsystem
  CnT : Subsystem
  Constant3 : Constant
  Divide2 : Product  Inputs=**/
  Divide3 : Product  Inputs=**/
  Divide4 : Product  Inputs=**/
  Gain1 : Gain  Gain=2
  Ground Effects : Subsystem  Commented=on
  Landing Gear Effects : Subsystem  Commented=on
  Mux1 : Mux
  Mux3 : Mux
  Terminator : Terminator  Commented=on
  Terminator1 : Terminator  Commented=on
  b(ft) : Constant  Value=ac.b
  cbar(ft) : Constant  Value=ac.cbar
  center of gravity as a fraction of cbar : Constant  Value=ac.x_cg
  r2d1 : Gain  Gain=1/25  SaturateOnIntegerOverflow=on  OutDataTypeStr=Inherit: Same as input  ParamDataTypeStr=Inherit: Same as input
  r2d2 : Gain  Gain=1/60  SaturateOnIntegerOverflow=on  OutDataTypeStr=Inherit: Same as input  ParamDataTypeStr=Inherit: Same as input
  r2d3 : Gain  Gain=1/20  SaturateOnIntegerOverflow=on  OutDataTypeStr=Inherit: Same as input  ParamDataTypeStr=Inherit: Same as input
  r2d4 : Gain  Gain=1/30  SaturateOnIntegerOverflow=on  OutDataTypeStr=Inherit: Same as input  ParamDataTypeStr=Inherit: Same as input
  reference center of gravity as a fraction of cbar : Constant  Value=ac.x_cg_ref
  CX_T : Outport  VectorParamsAs1DForOutWhenUnconnected=off
  CY_T : Outport  Port=2  VectorParamsAs1DForOutWhenUnconnected=off
  CZ_T : Outport  Port=3  VectorParamsAs1DForOutWhenUnconnected=off
  Cl_T_hat : Outport  Port=4  VectorParamsAs1DForOutWhenUnconnected=off
  Cm_T_hat : Outport  Port=5  VectorParamsAs1DForOutWhenUnconnected=off
  Cn_T_hat : Outport  Port=6  VectorParamsAs1DForOutWhenUnconnected=off
  gp : Outport  Port=7  VectorParamsAs1DForOutWhenUnconnected=off
  m_de : Outport  Port=8  VectorParamsAs1DForOutWhenUnconnected=off
  gr : Outport  Port=9  VectorParamsAs1DForOutWhenUnconnected=off
  wires:
  alpha (deg)/1 -> CXT/1(alpha (deg)), CYT/1(alpha (deg)), CmT/1(alpha (deg)), CnT/1(alpha (deg)), ClT/1(alpha (deg)), CZT/1(alpha (deg))
  beta (deg)/1 -> CXT/2(beta (deg)), CYT/2(beta (deg)), CZT/2(beta (deg)), ClT/2(beta (deg)), CmT/2(beta (deg)), CnT/2(beta (deg))
  elevator (deg)/1 -> CXT/3(elevator (deg)), CZT/3(elevator (deg)), ClT/3(elevator (deg)), CmT/3(elevator (deg)), CnT/3(elevator (deg))
  Vt (ft/s)/1 -> Gain1/1
  p (rad/s)/1 -> Divide4/1  "p"
  q (rad/s)/1 -> Divide2/1  "q"
  r (rad/s)/1 -> Divide3/1  "r"
  b(ft)/1 -> Divide4/2, Divide3/2, CnT/10(b)  "b"
  cbar(ft)/1 -> Divide2/2, CnT/9(cbar)  "cbar"
  Constant3/1 -> Add/1
  Add/1 -> CXT/4(dlef), CYT/3(dlef), CZT/4(dlef), ClT/4(dlef), CmT/4(dlef), CnT/4(dlef)  "dlef"
  alieron (deg)/1 -> r2d3/1
  rudder (deg)/1 -> r2d4/1
  Divide2/1 -> CZT/5(qc_2v), CXT/5(qc_2v), CmT/5(qc_2v)  "qc_2v"
  r2d3/1 -> CYT/4(dail)
  r2d4/1 -> CYT/5(drud)
  Divide3/1 -> CnT/5(rb_2v), ClT/5(rb_2v), CYT/6(rb_2v)  "rb_2v"
  Divide4/1 -> CnT/6(pb_2v), ClT/6(pb_2v), CYT/7(pb_2v)  "pb_2v"
  reference center of gravity as a fraction of cbar/1 -> CnT/7(x_cg_ref), CmT/6(x_cg_ref)
  center of gravity as a fraction of cbar/1 -> CnT/8(x_cg), CmT/7(x_cg)
  CZT/2(Cz_tot_plus) -> CmT/9(Cz_tot_plus)
  CZT/3(Cz_tot_minus) -> CmT/10(Cz_tot_minus)
  CYT/2(Cy_tot_n_mom) -> CnT/11(Cy_tot_n_mom)
  CYT/3(Cy_tot_n_da) -> CnT/12(Cy_tot_n_da)
  CYT/4(Cy_tot_n_dr) -> CnT/13(Cy_tot_n_dr)
  ClT/2(gp_da1) -> Mux1/1  "gp_da1"
  CnT/2(gp_da2) -> Mux1/2  "gp_da2"
  ClT/3(gp_dr1) -> Mux1/3  "gp_dr1"
  CnT/3(gp_dr2) -> Mux1/4  "gp_dr2"
  CmT/2(m_de) -> m_de/1  "m_de"
  ClT/4(gr_da1) -> Mux3/1  "gr_da1"
  CnT/4(gr_da2) -> Mux3/2  "gr_da2"
  ClT/5(gr_dr1) -> Mux3/3  "gr_dr1"
  CnT/5(gr_dr2) -> Mux3/4  "gr_dr2"
  SB (deg)/1 -> r2d2/1
  CXT/1(Cx_tot) -> CX_T/1
  CYT/1(Cy_tot) -> CY_T/1
  CZT/1(Cz_tot) -> CZ_T/1, CmT/8(Cz_tot)
  CnT/1(Cn_tot_hat) -> Cn_T_hat/1
  CmT/1(Cm_tot_hat) -> Cm_T_hat/1
  ClT/1(Cl_tot_hat) -> Cl_T_hat/1
  Mux1/1 -> gp/1
  Mux3/1 -> gr/1
  LEF (deg)/1 -> r2d1/1
  r2d1/1 -> Add/2
  r2d2/1 -> CXT/6(sb), CZT/6(sb), CmT/11(sb)
  Gain1/1 -> Divide3/3, Divide2/3, Divide4/3  "2v"
  Landing Gear Effects/1(Coeff) -> Terminator/1
  h_AGL/1 -> Ground Effects/3(h_AGL)
  Ground Effects/1(Coeff) -> Terminator1/1
  GearAngle/1 -> Landing Gear Effects/3(Landing Gear Angle)

== system example_main_NDI_f16/F-16 Vehicle Systems Model/Aerodynamic2/Creating    qbar // ps ==
  h (ft) : Inport
  Vt (ft/s) : Inport  Port=2
  Constant2 : Constant
  Constant3 : Constant  Value=390
  Constant6 : Constant  Value=4.14
  Math Function : Math  Operator=pow  SignedPower=on  SaturateOnIntegerOverflow=on
  Math Function1 : Math  Operator=square  SignedPower=on  SaturateOnIntegerOverflow=on
  Product : Product  Inputs=/*  InputSameDT=on  SaturateOnIntegerOverflow=on  OutDataTypeStr=Inherit: Same as first input
  Product5 : Product  Inputs=**  InputSameDT=on  SaturateOnIntegerOverflow=on  OutDataTypeStr=Inherit: Same as first input
  Product6 : Product  Inputs=**  InputSameDT=on  SaturateOnIntegerOverflow=on  OutDataTypeStr=Inherit: Same as first input
  Sum3 : Sum  Inputs=+-|  InputSameDT=on  SaturateOnIntegerOverflow=on  OutDataTypeStr=Inherit: Same as first input
  Switch : Switch  Threshold=35000  SaturateOnIntegerOverflow=on  InputSameDT=on
  r2d2 : Gain  Gain=0.703e-5  SaturateOnIntegerOverflow=on  OutDataTypeStr=Inherit: Same as input  ParamDataTypeStr=Inherit: Same as input
  r2d3 : Gain  Gain=519  SaturateOnIntegerOverflow=on  OutDataTypeStr=Inherit: Same as input  ParamDataTypeStr=Inherit: Same as input
  r2d4 : Gain  Gain=0.5  SaturateOnIntegerOverflow=on  OutDataTypeStr=Inherit: Same as input  ParamDataTypeStr=Inherit: Same as input
  r2d5 : Gain  Gain=1715  SaturateOnIntegerOverflow=on  OutDataTypeStr=Inherit: Same as input  ParamDataTypeStr=Inherit: Same as input
  rho0 : Gain  Gain=2.377e-3  SaturateOnIntegerOverflow=on  OutDataTypeStr=Inherit: Same as input  ParamDataTypeStr=Inherit: Same as input
  qbar / ps : Outport  VectorParamsAs1DForOutWhenUnconnected=off
  wires:
  h (ft)/1 -> r2d2/1, Switch/2
  Sum3/1 -> Math Function/1, r2d3/1  "tfac"
  Constant3/1 -> Switch/1
  r2d3/1 -> Switch/3
  Constant6/1 -> Math Function/2
  rho0/1 -> Product5/1, Product6/2  "rho"
  r2d2/1 -> Sum3/2
  Constant2/1 -> Sum3/1
  Math Function/1 -> rho0/1
  Math Function1/1 -> Product5/2
  Switch/1 -> r2d5/1  "temp"
  r2d5/1 -> Product6/1
  Product6/1 -> Product/1  "ps"
  Product5/1 -> r2d4/1  "qbar"
  Product/1 -> qbar / ps/1
  Vt (ft/s)/1 -> Math Function1/1  "Vt (ft/s)"
  r2d4/1 -> Product/2

== system example_main_NDI_f16/F-16 Vehicle Systems Model/Aerodynamic2/ISP  ==
  note: 1 T
      | 2 a (Speed of sound)
      | 3 P
      | 4 rho
      | 5 g
      | 6 mu (Coefficient of viscosity)
  h (ft) : Inport
  Vt (ft/s) : Inport  Port=2
  Demux : Demux  Outputs=[1,1,1,1,1,1]
      settings: DisplayOption=none
  Divide1 : Product  Inputs=*/
  Length Conversion : aerolibconvert2/Length Conversion  IU=ft  OU=m
  MATLAB Function : MATLAB Function  TreatAsAtomicUnit=on
  Product : Product
  Square : Math  Operator=square  SignedPower=on  SaturateOnIntegerOverflow=on
  r2d1 : Gain  Gain=0.5  SaturateOnIntegerOverflow=on  OutDataTypeStr=Inherit: Same as input  ParamDataTypeStr=Inherit: Same as input
  r2d3 : Gain  Gain=3.2808399  SaturateOnIntegerOverflow=on  OutDataTypeStr=Inherit: Same as input  ParamDataTypeStr=Inherit: Same as input
  r2d4 : Gain  Gain=0.00194032033  SaturateOnIntegerOverflow=on  OutDataTypeStr=Inherit: Same as input  ParamDataTypeStr=Inherit: Same as input
  T(K) : Outport  VectorParamsAs1DForOutWhenUnconnected=off
  "Mach " : Outport  Port=2  VectorParamsAs1DForOutWhenUnconnected=off
  P(HPa) : Outport  Port=3  VectorParamsAs1DForOutWhenUnconnected=off
  "qbar " : Outport  Port=4  VectorParamsAs1DForOutWhenUnconnected=off
  rho : Outport  Port=5  VectorParamsAs1DForOutWhenUnconnected=off
  g (m/s^2) : Outport  Port=6  VectorParamsAs1DForOutWhenUnconnected=off
  mu : Outport  Port=7  VectorParamsAs1DForOutWhenUnconnected=off
  wires:
  r2d3/1 -> Divide1/2
  r2d1/1 -> Product/2
  Demux/4 -> rho/1, r2d4/1  "rho(kg/m^3)"
  Demux/2 -> r2d3/1  "a(m/s)"
  Demux/1 -> T(K)/1  "T(K)"
  r2d4/1 -> r2d1/1
  Divide1/1 -> "Mach "/1
  Demux/5 -> g (m/s^2)/1  "g (m/s^2)"
  Demux/6 -> mu/1  "mu"
  Product/1 -> "qbar "/1
  Square/1 -> Product/1
  Vt (ft/s)/1 -> Square/1, Divide1/1
  Demux/3 -> P(HPa)/1  "P(Pa)"
  h (ft)/1 -> Length Conversion/1
  Length Conversion/1 -> MATLAB Function/1(h)
  MATLAB Function/1(ISP_output) -> Demux/1

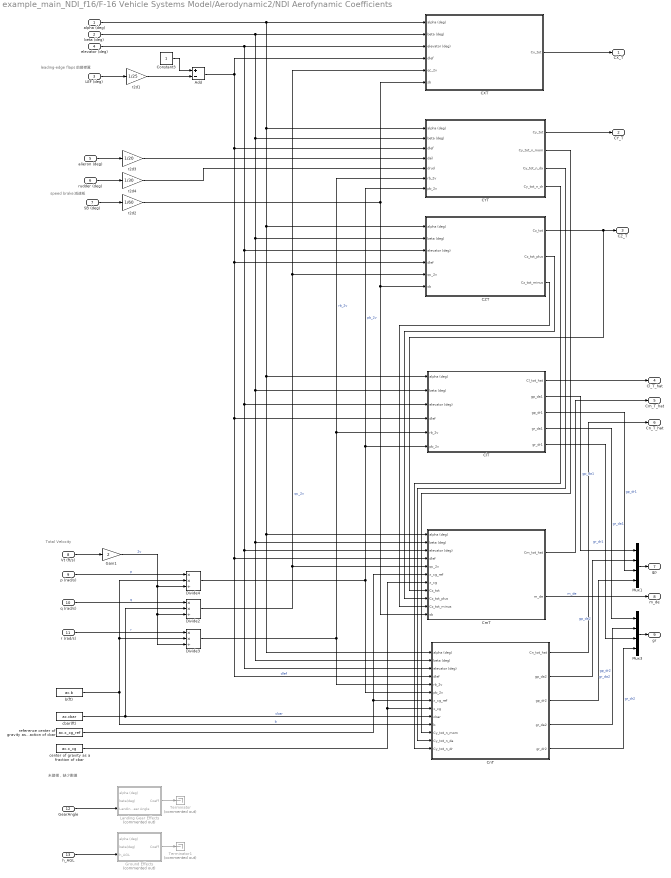
== system example_main_NDI_f16/F-16 Vehicle Systems Model/Aerodynamic2/NDI Aerofynamic Coefficients ==
  note: leading-edge flaps
      | 前緣襟翼
  note: speed brake
      | 減速板
  note: Total Velocity
  note: 未建模，缺少數據
  alpha (deg) : Inport
  beta (deg) : Inport  Port=2
  LEF (deg) : Inport  Port=3
  elevator (deg) : Inport  Port=4
  alieron (deg) : Inport  Port=5
  rudder (deg) : Inport  Port=6
  SB (deg) : Inport  Port=7  Unit=deg
  Vt (ft/s) : Inport  Port=8
  p (rad/s) : Inport  Port=9
  q (rad/s) : Inport  Port=10
  r (rad/s) : Inport  Port=11
  GearAngle : Inport  Port=12
  h_AGL : Inport  Port=13
  Add : Sum  Inputs=+-
  CXT : Subsystem
  CYT : Subsystem
  CZT : Subsystem
  ClT : Subsystem
  CmT : Subsystem
  CnT : Subsystem
  Constant3 : Constant
  Divide2 : Product  Inputs=**/
  Divide3 : Product  Inputs=**/
  Divide4 : Product  Inputs=**/
  Gain1 : Gain  Gain=2
  Ground Effects : Subsystem  Commented=on
  Landing Gear Effects : Subsystem  Commented=on
  Mux1 : Mux
  Mux3 : Mux
  Terminator : Terminator  Commented=on
  Terminator1 : Terminator  Commented=on
  b(ft) : Constant  Value=ac.b
  cbar(ft) : Constant  Value=ac.cbar
  center of gravity as a fraction of cbar : Constant  Value=ac.x_cg
  r2d1 : Gain  Gain=1/25  SaturateOnIntegerOverflow=on  OutDataTypeStr=Inherit: Same as input  ParamDataTypeStr=Inherit: Same as input
  r2d2 : Gain  Gain=1/60  SaturateOnIntegerOverflow=on  OutDataTypeStr=Inherit: Same as input  ParamDataTypeStr=Inherit: Same as input
  r2d3 : Gain  Gain=1/20  SaturateOnIntegerOverflow=on  OutDataTypeStr=Inherit: Same as input  ParamDataTypeStr=Inherit: Same as input
  r2d4 : Gain  Gain=1/30  SaturateOnIntegerOverflow=on  OutDataTypeStr=Inherit: Same as input  ParamDataTypeStr=Inherit: Same as input
  reference center of gravity as a fraction of cbar : Constant  Value=ac.x_cg_ref
  CX_T : Outport  VectorParamsAs1DForOutWhenUnconnected=off
  CY_T : Outport  Port=2  VectorParamsAs1DForOutWhenUnconnected=off
  CZ_T : Outport  Port=3  VectorParamsAs1DForOutWhenUnconnected=off
  Cl_T_hat : Outport  Port=4  VectorParamsAs1DForOutWhenUnconnected=off
  Cm_T_hat : Outport  Port=5  VectorParamsAs1DForOutWhenUnconnected=off
  Cn_T_hat : Outport  Port=6  VectorParamsAs1DForOutWhenUnconnected=off
  gp : Outport  Port=7  VectorParamsAs1DForOutWhenUnconnected=off
  m_de : Outport  Port=8  VectorParamsAs1DForOutWhenUnconnected=off
  gr : Outport  Port=9  VectorParamsAs1DForOutWhenUnconnected=off
  wires:
  alpha (deg)/1 -> CXT/1(alpha (deg)), CYT/1(alpha (deg)), CmT/1(alpha (deg)), CnT/1(alpha (deg)), ClT/1(alpha (deg)), CZT/1(alpha (deg))
  beta (deg)/1 -> CXT/2(beta (deg)), CYT/2(beta (deg)), CZT/2(beta (deg)), ClT/2(beta (deg)), CmT/2(beta (deg)), CnT/2(beta (deg))
  elevator (deg)/1 -> CXT/3(elevator (deg)), CZT/3(elevator (deg)), ClT/3(elevator (deg)), CmT/3(elevator (deg)), CnT/3(elevator (deg))
  Vt (ft/s)/1 -> Gain1/1
  p (rad/s)/1 -> Divide4/1  "p"
  q (rad/s)/1 -> Divide2/1  "q"
  r (rad/s)/1 -> Divide3/1  "r"
  b(ft)/1 -> Divide4/2, Divide3/2, CnT/10(b)  "b"
  cbar(ft)/1 -> Divide2/2, CnT/9(cbar)  "cbar"
  Constant3/1 -> Add/1
  Add/1 -> CXT/4(dlef), CYT/3(dlef), CZT/4(dlef), ClT/4(dlef), CmT/4(dlef), CnT/4(dlef)  "dlef"
  alieron (deg)/1 -> r2d3/1
  rudder (deg)/1 -> r2d4/1
  Divide2/1 -> CZT/5(qc_2v), CXT/5(qc_2v), CmT/5(qc_2v)  "qc_2v"
  r2d3/1 -> CYT/4(dail)
  r2d4/1 -> CYT/5(drud)
  Divide3/1 -> CnT/5(rb_2v), ClT/5(rb_2v), CYT/6(rb_2v)  "rb_2v"
  Divide4/1 -> CnT/6(pb_2v), ClT/6(pb_2v), CYT/7(pb_2v)  "pb_2v"
  reference center of gravity as a fraction of cbar/1 -> CnT/7(x_cg_ref), CmT/6(x_cg_ref)
  center of gravity as a fraction of cbar/1 -> CnT/8(x_cg), CmT/7(x_cg)
  CZT/2(Cz_tot_plus) -> CmT/9(Cz_tot_plus)
  CZT/3(Cz_tot_minus) -> CmT/10(Cz_tot_minus)
  CYT/2(Cy_tot_n_mom) -> CnT/11(Cy_tot_n_mom)
  CYT/3(Cy_tot_n_da) -> CnT/12(Cy_tot_n_da)
  CYT/4(Cy_tot_n_dr) -> CnT/13(Cy_tot_n_dr)
  ClT/2(gp_da1) -> Mux1/1  "gp_da1"
  CnT/2(gp_da2) -> Mux1/2  "gp_da2"
  ClT/3(gp_dr1) -> Mux1/3  "gp_dr1"
  CnT/3(gp_dr2) -> Mux1/4  "gp_dr2"
  CmT/2(m_de) -> m_de/1  "m_de"
  ClT/4(gr_da1) -> Mux3/1  "gr_da1"
  CnT/4(gr_da2) -> Mux3/2  "gr_da2"
  ClT/5(gr_dr1) -> Mux3/3  "gr_dr1"
  CnT/5(gr_dr2) -> Mux3/4  "gr_dr2"
  SB (deg)/1 -> r2d2/1
  CXT/1(Cx_tot) -> CX_T/1
  CYT/1(Cy_tot) -> CY_T/1
  CZT/1(Cz_tot) -> CZ_T/1, CmT/8(Cz_tot)
  CnT/1(Cn_tot_hat) -> Cn_T_hat/1
  CmT/1(Cm_tot_hat) -> Cm_T_hat/1
  ClT/1(Cl_tot_hat) -> Cl_T_hat/1
  Mux1/1 -> gp/1
  Mux3/1 -> gr/1
  LEF (deg)/1 -> r2d1/1
  r2d1/1 -> Add/2
  r2d2/1 -> CXT/6(sb), CZT/6(sb), CmT/11(sb)
  Gain1/1 -> Divide3/3, Divide2/3, Divide4/3  "2v"
  Landing Gear Effects/1(Coeff) -> Terminator/1
  h_AGL/1 -> Ground Effects/3(h_AGL)
  Ground Effects/1(Coeff) -> Terminator1/1
  GearAngle/1 -> Landing Gear Effects/3(Landing Gear Angle)

== system example_main_NDI_f16/F-16 Vehicle Systems Model/Vehicle/6DOF (Quaternion) ==
  note: TODO: 改成旋轉矩陣相乘、輸出座標轉換 旋轉矩陣
  note: 1 npos
      | 2 epos
      | 3 alt
      | 4 q0
      | 5 q1
      | 6 q2
      | 7 q3
      | 8 P
      | 9 Q
      | 10 R
      | 11 alpha
      | 12 beta
      | 13 mu
      | 14 vt
      | 15 chi
      | 16 gamma
      | ------------------------
      | X 17 Tx
      | X 18 Ty
      | X 19 Tz
      | X 20 Mx_T
      | X 21 My_T
      | X 22 Mz_T
      | X 23 T
      | --------------------
      | X 24 ele
      | X 25 ail
      | X 26 rud
      | -------------------
      | X 27 delta_z
      | X 28 delta_y
      | -----------------
      | X 29 qbar
      | -----------------
      | X 30 CXT
      | X 31 CYT
      | X 32 CZT
      | X 33 CLT
      | X 34 CMT
      | X 35 CNT
      | -----------------
      | X 36 lef
  note: 1 npos
      | 2 epos
      | 3 alt
      | 4 q0
      | 5 q1
      | 6 q2
      | 7 q3
      | 8 P
      | 9 Q
      | 10 R
      | 11 alpha
      | 12 beta
      | 13 mu
      | 14 vt
      | 15 chi
      | 16 gamma
  note: Note：
      |
      | 宥瑋論文6.4.3節、附錄B響應圖初始值
      | [0 0 -1000 0.9963 0 0.086 0  0 0 0 deg2rad(9.8641) 0 0 287 0 0]
  Fxyz : Inport
  Mxyz : Inport  Port=2
  AeroFM : Inport  Port=3
  Txyz : Inport  Port=4
  gravity : Inport  Port=5
  Demux : Demux  Outputs=16
      settings: DisplayOption=none
  Demux3 : Demux  Outputs=3
  Demux4 : Demux  Outputs=8
  Integrator : Integrator  InitialCondition=state0
  Ix(slug*ft^2) : Constant  Value=ac.Ix
  Ixz(slug*ft^2)1 : Constant  Value=ac.Ixz
  Iy(slug*ft^2) : Constant  Value=ac.Iy
  Iz(slug*ft^2) : Constant  Value=ac.Iz
  MATLAB Function : MATLAB Function  TreatAsAtomicUnit=on
  MATLAB Function2 : MATLAB Function  TreatAsAtomicUnit=on
  Mux1 : Mux  Inputs=[1,1,1,1]
  Quateration : MATLAB Function  TreatAsAtomicUnit=on
  Quaternion Normalization : Subsystem
  Selector : Selector  InputPortWidth=16  IndexOptions=Index vector (dialog)  Indices=[11 12 14]  OutputSizes=3
  Selector1 : Selector  InputPortWidth=16  IndexOptions=Index vector (dialog)  Indices=[8:14 16]  OutputSizes=3
  mass (slugs) : Constant  Value=ac.m
  turbine momentum along roll axis (slug*ft^2) : Constant  Value=ac.Heng
  npos : Outport  VectorParamsAs1DForOutWhenUnconnected=off
  epos : Outport  Port=2  VectorParamsAs1DForOutWhenUnconnected=off
  altitude : Outport  Port=3  VectorParamsAs1DForOutWhenUnconnected=off
  q0q1q2q3 : Outport  Port=4
  p : Outport  Port=5  VectorParamsAs1DForOutWhenUnconnected=off
  q : Outport  Port=6  VectorParamsAs1DForOutWhenUnconnected=off
  r : Outport  Port=7  VectorParamsAs1DForOutWhenUnconnected=off
  alpha : Outport  Port=8  VectorParamsAs1DForOutWhenUnconnected=off
  beta : Outport  Port=9  VectorParamsAs1DForOutWhenUnconnected=off
  mu : Outport  Port=10  VectorParamsAs1DForOutWhenUnconnected=off
  Vt : Outport  Port=11  VectorParamsAs1DForOutWhenUnconnected=off
  chi : Outport  Port=12  VectorParamsAs1DForOutWhenUnconnected=off
  gamma : Outport  Port=13  VectorParamsAs1DForOutWhenUnconnected=off
  phi : Outport  Port=14  VectorParamsAs1DForOutWhenUnconnected=off
  theta : Outport  Port=15  VectorParamsAs1DForOutWhenUnconnected=off
  psi : Outport  Port=16  VectorParamsAs1DForOutWhenUnconnected=off
  an : Outport  Port=17
  ay : Outport  Port=18
  wires:
  Demux/2 -> epos/1  "epos"
  Demux/3 -> altitude/1  "altitude"
  Integrator/1 -> MATLAB Function/1(xu), Selector1/1, Demux/1
  MATLAB Function/1(dxdt) -> Integrator/1, Selector/1
  Demux/1 -> npos/1  "npos"
  Demux/5 -> Mux1/2  "q1"
  Demux/4 -> Mux1/1  "q0"
  Demux/7 -> Mux1/4  "q3"
  Demux/6 -> Mux1/3  "q2"
  Demux/8 -> p/1  "p"
  Demux/9 -> q/1  "q"
  Demux/10 -> r/1  "r"
  Demux/11 -> alpha/1  "alpha"
  Demux/12 -> beta/1  "beta"
  Demux/13 -> mu/1  "mu"
  Demux/14 -> Vt/1  "Vt"
  Demux/15 -> chi/1  "chi"
  Demux/16 -> gamma/1  "gamma"
  Mux1/1 -> Quaternion Normalization/1(q)
  Quaternion Normalization/1(qnorm) -> q0q1q2q3/1, Quateration/1(Q)  "q0q1q2q3"
  AeroFM/1 -> MATLAB Function/4(AeroFM)
  Mxyz/1 -> MATLAB Function/3(Mxyz)
  Fxyz/1 -> MATLAB Function/2(Fxyz)
  Txyz/1 -> MATLAB Function/5(Txyz)
  gravity/1 -> MATLAB Function2/12(g), MATLAB Function/12(g)
  Ix(slug*ft^2)/1 -> MATLAB Function/7(Ix)
  Iy(slug*ft^2)/1 -> MATLAB Function/8(Iy)
  Iz(slug*ft^2)/1 -> MATLAB Function/9(Iz)
  Ixz(slug*ft^2)1/1 -> MATLAB Function/10(Ixz)
  turbine momentum along roll axis (slug*ft^2)/1 -> MATLAB Function/11(Heng)
  mass (slugs)/1 -> MATLAB Function/6(m)
  Quateration/1(phi) -> phi/1
  Quateration/2(theta) -> theta/1
  Quateration/3(psi) -> psi/1
  Selector/1 -> Demux3/1
  Demux3/1 -> MATLAB Function2/9(alpha_dot)
  Demux3/2 -> MATLAB Function2/10(beta_dot)
  Demux3/3 -> MATLAB Function2/11(Vt_dot)
  Selector1/1 -> Demux4/1
  Demux4/1 -> MATLAB Function2/1(p)
  Demux4/2 -> MATLAB Function2/2(q)
  Demux4/3 -> MATLAB Function2/3(r)
  Demux4/4 -> MATLAB Function2/4(alpha)
  Demux4/5 -> MATLAB Function2/5(beta)
  Demux4/6 -> MATLAB Function2/6(mu)
  Demux4/7 -> MATLAB Function2/7(vt)
  Demux4/8 -> MATLAB Function2/8(gamma)
  MATLAB Function2/1(an) -> an/1
  MATLAB Function2/2(ay) -> ay/1
